simulink subsystem "SSCFuelCell"  (R2025b)
settings: Solver=VariableStepAuto  StartTime=0.0  StopTime=10.0  RelTol=1e-3
undefined symbols (not defined in the file): anode_tube_D, cathode_tube_D, comp_rpm_TLU, coolant_num_layers, coolant_num_passes, coolant_tube_D, coolant_w_channels, env_p, env_T, f_fc_voltage, N2_T, radiator_air_area_fins, radiator_air_area_primary, radiator_eta_fin, radiator_N_tubes, radiator_rho, radiator_t_wall, radiator_tube_H, radiator_W, stack_area, stack_iL, stack_mea_rho, stack_num_cells, stack_num_channels, stack_t_gdl, stack_t_membrane, stack_w_channels
libraries: fl_lib x100, nesl_utility x20, slpidlib x2
(part 3 of 3)

== system SSCFuelCell/Recirculation ==
  Constant Volume Chamber (MA) : fl_lib/Moist Air/Elements/Constant Volume Chamber (MA)  volume=0.05^3 m^3  num_ports=foundation.enum.num_ports.three  area_A=pi*anode_tube_D^2/4 m^2  area_B=pi*anode_tube_D^2/4 m^2  area_C=pi*anode_tube_D^2/4 m^2  area_D=0.01 m^2  RH_ws=1  time_constant_cond=1e-3 s  time_constant_evap=1e-3 s  fraction_entrained=1  moisture_trace_gas_source=foundation.enum.moisture_trace_gas_source.none  moisture_source_spec=foundation.enum.MoistureSourceSpec.WaterVapor  vapor_from_liquid=false  moisture_mass_flow=0 kg/s  moisture_temperature_spec=foundation.enum.temperature_spec.atmospheric  moisture_temperature=293.15 K  trace_gas_mass_flow=0 kg/s  trace_gas_temperature_spec=foundation.enum.temperature_spec.atmospheric  trace_gas_temperature=293.15 K  p_init=env_p MPa  p_init_priority=foundation.enum.Priority.High  T_init=env_T degC  T_init_priority=foundation.enum.Priority.High  humidity_spec=foundation.enum.HumiditySpec.RelativeHumidity  RH_init=0  RH_init_priority=foundation.enum.Priority.High  x_w_init=0  x_w_init_priority=foundation.enum.Priority.None  y_w_init=0  y_w_init_priority=foundation.enum.Priority.None  HR_init=0  HR_init_priority=foundation.enum.Priority.None  Tw_init=287 K  Tw_init_priority=foundation.enum.Priority.High  trace_gas_spec=foundation.enum.trace_gas_spec.mole_fraction  x_g_init=0  x_g_init_priority=foundation.enum.Priority.None  y_g_init=tank_yH2  y_g_init_priority=foundation.enum.Priority.High  r_d_init=0  r_d_init_priority=foundation.enum.Priority.High
      settings: InternalSimscapePortConfiguration="{\"Bottom\":[],\"Left\":[{\"id\":\"A\",\"label\":\"A\",\"type\":\"foundation.moist_air.moist_air\"},{\"id\":\"B\",\"label\":\"B\",\"type\":\"foundation.moist_air.moist_air\"},{\"id\":\"C\",\"label\":\"C\",\"type\":\"foundation.moist_air.moist_air\"}],\"Right\":[{\"id\":\"W\",\"label\":\"W\",\"type\":\"output\"},{\"id\":\"F\",\"label\":\"F\",\"type\":\"output\"},{\"id\":\"H\",\"label\":\"H\",\"type\":\"foundation.thermal.thermal\"}],\"Top\":[]}"
  Controlled Mass Flow Rate Source (MA) : fl_lib/Moist Air/Sources/Flow Rate Source (MA)  source_type=foundation.enum.constant_controlled.controlled  flow_type=foundation.enum.mass_volumetric_flow.mass  mass_flow=0 kg/s  volumetric_flow=0 m^3/s  volumetric_flow_conditions=foundation.enum.volumetric_flow_conditions.actual  p_std=0.101325 MPa  T_std=20 degC  RH_std=0.65  power_spec=foundation.enum.power_spec.isentropic  area_A=pi*anode_tube_D^2/4 m^2  area_B=pi*anode_tube_D^2/4 m^2
      settings: InternalSimscapePortConfiguration="{\"Bottom\":[],\"Left\":[{\"id\":\"A\",\"label\":\"A\",\"type\":\"foundation.moist_air.moist_air\"},{\"id\":\"M\",\"label\":\"M\",\"type\":\"input\"}],\"Right\":[{\"id\":\"B\",\"label\":\"B\",\"type\":\"foundation.moist_air.moist_air\"}],\"Top\":[]}"
  Feedforward Control : Subsystem
  Max Flow : fl_lib/Physical Signals/Functions/PS Gain  gain=0.01 kg/s
  Perfect Insulator : fl_lib/Thermal/Thermal Elements/Perfect Insulator  T_specify=off  T_priority=None  T=0 K  T_nominal_specify=off  T_nominal_value=1  T_nominal_unit=K
  Simulink-PS Converter : nesl_utility/Simulink-PS Converter  PhysicalDomain=network_engine_domain  SubClassName=ps_input  LeftPortType=input  RightPortType=output  PseudoPeriodic=off  Frequencies=[]  NoiseDistribution=none  NoiseParameters=[]  Unit=1  AffineConversion=off  FilteringAndDerivatives=provide  SimscapeFilterOrder=1  InputFilterTimeConstant=0.001  UdotUserProvided=0
  A : PMIOPort  Side=Left
  B : PMIOPort  Port=2  Side=Right
  R : PMIOPort  Port=3  Side=Right
  wires:
  [i_stack] -> Feedforward Control/1(i)
  Feedforward Control/1(cmd) -> Simulink-PS Converter/1
  connections:
  Perfect Insulator/LConn1 -- Constant Volume Chamber (MA)/RConn3
  Controlled Mass Flow Rate Source (MA)/RConn1 -- Constant Volume Chamber (MA)/LConn2
  A/RConn1 -- Constant Volume Chamber (MA)/LConn1
  B/RConn1 -- Constant Volume Chamber (MA)/LConn3
  R/RConn1 -- Controlled Mass Flow Rate Source (MA)/LConn1
  Max Flow/RConn1 -- Controlled Mass Flow Rate Source (MA)/LConn2
  Simulink-PS Converter/RConn1 -- Max Flow/LConn1

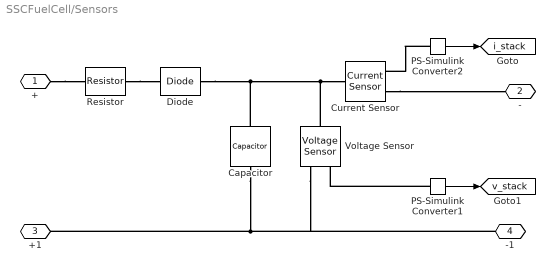
== system SSCFuelCell/Sensors ==
  Capacitor : fl_lib/Electrical/Electrical Elements/Capacitor  c=1e-6 F  r=1e-6 Ohm  g=0 1/Ohm  i_specify=off  i_priority=None  i=0 A  i_nominal_specify=off  i_nominal_value=1  i_nominal_unit=A  v_specify=off  v_priority=None  v=0 V  v_nominal_specify=off  v_nominal_value=1  v_nominal_unit=V  vc_specify=on  vc_priority=High  vc=f_fc_voltage(1) V  vc_nominal_specify=off  vc_nominal_value=1  vc_nominal_unit=V
  Current Sensor : fl_lib/Electrical/Electrical Sensors/Current Sensor
  Diode : fl_lib/Electrical/Electrical Elements/Diode  Vf=0.6 V  Ron=0.3 Ohm  Goff=1e-8 1/Ohm  i_specify=off  i_priority=None  i=0 A  i_nominal_specify=off  i_nominal_value=1  i_nominal_unit=A  v_specify=off  v_priority=None  v=0 V  v_nominal_specify=off  v_nominal_value=1  v_nominal_unit=V
  PS-Simulink Converter1 : nesl_utility/PS-Simulink Converter  PhysicalDomain=network_engine_domain  SubClassName=ps_output  LeftPortType=input  RightPortType=output  PseudoPeriodic=off  Frequencies=[]  VectorFormat=1-D array  Unit=V  AffineConversion=off
  PS-Simulink Converter2 : nesl_utility/PS-Simulink Converter  PhysicalDomain=network_engine_domain  SubClassName=ps_output  LeftPortType=input  RightPortType=output  PseudoPeriodic=off  Frequencies=[]  VectorFormat=1-D array  Unit=A  AffineConversion=off
  Resistor : fl_lib/Electrical/Electrical Elements/Resistor  R=1e-3 Ohm  i_specify=off  i_priority=None  i=0 A  i_nominal_specify=off  i_nominal_value=1  i_nominal_unit=A  v_specify=off  v_priority=None  v=0 V  v_nominal_specify=off  v_nominal_value=1  v_nominal_unit=V
  Voltage Sensor : fl_lib/Electrical/Electrical Sensors/Voltage Sensor
  + : PMIOPort  Side=Left
  - : PMIOPort  Port=2  Side=Right
  +1 : PMIOPort  Port=3  Side=Left
  -1 : PMIOPort  Port=4  Side=Right
  tag scope: i_stack=global, v_stack=global
  wires:
  PS-Simulink Converter1/1 -> [v_stack]
  PS-Simulink Converter2/1 -> [i_stack]
  connections:
  Capacitor/RConn1 -- -1/RConn1 -- Voltage Sensor/RConn2 -- +1/RConn1
  Capacitor/LConn1 -- Diode/RConn1 -- Current Sensor/LConn1 -- Voltage Sensor/LConn1
  +/RConn1 -- Resistor/LConn1
  Current Sensor/RConn2 -- -/RConn1
  PS-Simulink Converter1/LConn1 -- Voltage Sensor/RConn1
  Resistor/RConn1 -- Diode/LConn1
  PS-Simulink Converter2/LConn1 -- Current Sensor/RConn1

== system SSCFuelCell/Anode Humidifier/Proportional Control ==
  RH_set : Inport
  RH_meas : Inport  Port=2
  Gain : Gain  Gain=0.1
  Saturation : Saturate  UpperLimit=inf  LowerLimit=0  ZeroCross=off
  Sum : Sum  Inputs=|+-
  Transfer Fcn : TransferFcn  Denominator=[1 1]
  Mw : Outport
  wires:
  Saturation/1 -> Transfer Fcn/1
  RH_meas/1 -> Sum/2
  RH_set/1 -> Sum/1
  Sum/1 -> Gain/1
  Gain/1 -> Saturation/1
  Transfer Fcn/1 -> Mw/1

== system SSCFuelCell/Cathode Humidifier/Proportional Control ==
  RH_set : Inport
  RH_meas : Inport  Port=2
  Gain : Gain  Gain=0.1
  Saturation : Saturate  UpperLimit=inf  LowerLimit=0  ZeroCross=off
  Sum : Sum  Inputs=|+-
  Transfer Fcn : TransferFcn  Denominator=[1 1]
  Mw : Outport
  wires:
  Saturation/1 -> Transfer Fcn/1
  Gain/1 -> Saturation/1
  Transfer Fcn/1 -> Mw/1
  RH_meas/1 -> Sum/2
  Sum/1 -> Gain/1
  RH_set/1 -> Sum/1

== system SSCFuelCell/Cathode Exhaust/Pressure Relief Valve ==
  Absolute Reference (MA) : fl_lib/Moist Air/Elements/Absolute Reference (MA)
  PS Add : fl_lib/Physical Signals/Functions/PS Add
  PS Constant : fl_lib/Physical Signals/Sources/PS Constant  constant=r_min^2
  PS Gain : fl_lib/Physical Signals/Functions/PS Gain  gain=(r_max^2 - r_min^2)/p_range 1/MPa
  PS Gain1 : fl_lib/Physical Signals/Functions/PS Gain  gain=pi*D^2/4 m^2
  PS Subtract : fl_lib/Physical Signals/Functions/PS Subtract
  Pressure & Temperature Sensor (MA) : fl_lib/Moist Air/Sensors/Pressure & Temperature Sensor (MA)  reference=foundation.enum.MeasurementReference.difference  pressure=true  pressure_spec=foundation.enum.PressureMeasementSpec.Absolute  temperature=true
      settings: InternalSimscapePortConfiguration="{\"Bottom\":[{\"id\":\"T\",\"label\":\"T\",\"type\":\"output\"}],\"Left\":[{\"id\":\"A\",\"label\":\"A\",\"type\":\"foundation.moist_air.moist_air\"}],\"Right\":[{\"id\":\"B\",\"label\":\"B\",\"type\":\"foundation.moist_air.moist_air\"},{\"id\":\"P\",\"label\":\"P\",\"type\":\"output\"}],\"Top\":[]}"
  Valve : fl_lib/Moist Air/Elements/Local Restriction (MA)  restriction_type=foundation.enum.restriction_type.variable  restriction_area=0.001 m^2  min_area=pi*(r_min*D)^2/4 m^2  max_area=pi*(r_max*D)^2/4 m^2  area=pi*D^2/4 m^2  Cd=0.64  B_lam=0.999
  A : PMIOPort  Side=Left
  B : PMIOPort  Port=2  Side=Right
  p_set : PMIOPort  Port=3  Side=Left
  connections:
  PS Add/RConn1 -- PS Gain1/LConn1
  PS Gain/LConn1 -- PS Subtract/RConn1
  PS Gain1/RConn1 -- Valve/LConn2
  Absolute Reference (MA)/LConn1 -- Pressure & Temperature Sensor (MA)/RConn1
  Valve/RConn1 -- B/RConn1
  Valve/LConn1 -- A/RConn1 -- Pressure & Temperature Sensor (MA)/LConn1
  PS Gain/RConn1 -- PS Add/LConn1
  PS Add/LConn2 -- PS Constant/RConn1
  Pressure & Temperature Sensor (MA)/RConn2 -- PS Subtract/LConn1
  p_set/RConn1 -- PS Subtract/LConn2

== system SSCFuelCell/Cooling System/Coolant Tank ==
  Coolant Volume : fl_lib/Thermal Liquid/Elements/Translational Mechanical Converter (TL)  mech_orientation=foundation.enum.MechOrientationTranslational.Positive  displacement_spec=foundation.enum.DisplacementSpec.Calculate  x0=x_init m  interface_area=A m^2  dead_volume=A * 0.001 m^3  environment_spec=foundation.enum.pressure_spec.atmospheric  environment_pressure=0.101325 MPa  dynamic_compressibility=simscape.enum.onoff.off  p0=env_p MPa  T0=env_T degC  p_nominal=0.101325 MPa  T_nominal=293.15 K
      settings: InternalSimscapePortConfiguration="{\"Bottom\":[],\"Left\":[{\"id\":\"A\",\"label\":\"A\",\"type\":\"foundation.thermal_liquid.thermal_liquid\"},{\"id\":\"C\",\"label\":\"C\",\"type\":\"foundation.mechanical.translational.translational\"},{\"id\":\"H\",\"label\":\"H\",\"type\":\"foundation.thermal.thermal\"}],\"Right\":[{\"id\":\"R\",\"label\":\"R\",\"type\":\"foundation.mechanical.translational.translational\"}],\"Top\":[]}"
  Mechanical Translational Reference : fl_lib/Mechanical/Translational Elements/Mechanical Translational Reference
  Perfect Insulator : fl_lib/Thermal/Thermal Elements/Perfect Insulator  T_specify=off  T_priority=None  T=0 K  T_nominal_specify=off  T_nominal_value=1  T_nominal_unit=K
  Translational Free End : fl_lib/Mechanical/Translational Elements/Translational Free End  v_specify=off  v_priority=None  v=0 m/s  v_nominal_specify=off  v_nominal_value=1  v_nominal_unit=m/s
      settings: InternalSimscapePortConfiguration="{\"Bottom\":[],\"Left\":[{\"id\":\"V\",\"label\":\"\",\"type\":\"foundation.mechanical.translational.translational\"}],\"Right\":[],\"Top\":[]}"
  T : PMIOPort  Side=Right
  connections:
  Coolant Volume/LConn1 -- T/RConn1
  Mechanical Translational Reference/LConn1 -- Coolant Volume/LConn2
  Translational Free End/LConn1 -- Coolant Volume/RConn1
  Perfect Insulator/LConn1 -- Coolant Volume/LConn3

== system SSCFuelCell/Cooling System/Pump Control ==
  T_set : Inport
  T_meas : Inport  Port=2
  Control Signals : Scope  NumInputPorts=2
      settings: Title=Stack Temperature (degC)  ActiveDisplayYMinimum=12.33618  ActiveDisplayYMaximum=88.97437
  Mux : Mux  Inputs=2
  Mux1 : Mux  Inputs=2
  PID Controller : slpidlib/PID Controller  Controller=PI  Form=Ideal  TimeDomain=Continuous-time  UseExternalTs=off  SampleTime=-1  IntegratorMethod=Forward Euler  FilterMethod=Forward Euler  ControllerParametersSource=internal  P=0.1  I=0.01  UseKiTs=off  D=0  UseExternalDerivativeSource=off  N=100  UseFilter=on  TunerSelectOption=Transfer Function Based (PID Tuner App)  InitialConditionSource=internal  InitialConditionForIntegrator=0  InitialConditionForFilter=0  DifferentiatorICPrevScaledInput=0  ExternalReset=none  TrackingMode=off  Kt=1  LimitOutput=on  SatLimitsSource=internal  UpperSaturationLimit=1  LowerSaturationLimit=0  LinearizeAsGain=on  AntiWindupMode=back-calculation  Kb=0.1  LimitIntegrator=off  UpperIntegratorSaturationLimit=inf  LowerIntegratorSaturationLimit=-inf  POutMin=[]  POutMax=[]  IOutMin=[]  IOutMax=[]  DOutMin=[]  DOutMax=[]  NOutMin=[]  NOutMax=[]  SumOutMin=[]  SumOutMax=[]  SaturationOutMin=[]  SaturationOutMax=[]  PParamMin=[]  PParamMax=[]  IParamMin=[]  IParamMax=[]  DParamMin=[]  DParamMax=[]  NParamMin=[]  NParamMax=[]  KbParamMin=[]  KbParamMax=[]  KtParamMin=[]  KtParamMax=[]  KbOutMin=[]  KbOutMax=[]  KtOutMin=[]  KtOutMax=[]  IntegratorOutMin=[]  IntegratorOutMax=[]  FilterOutMin=[]  FilterOutMax=[]  SumI1OutMin=[]  SumI1OutMax=[]  SumI2OutMin=[]  SumI2OutMax=[]  SumI3OutMin=[]  SumI3OutMax=[]  SumI4OutMin=[]  SumI4OutMax=[]  SumDOutMin=[]  SumDOutMax=[]  DifferentiatorOutMin=[]  DifferentiatorOutMax=[]  FilterDiffOutCoefMin=[]  FilterDiffOutCoefMax=[]  ReciprocalOutMin=[]  ReciprocalOutMax=[]  SumDenOutMin=[]  SumDenOutMax=[]  SumNumOutMin=[]  SumNumOutMax=[]  DivideOutMin=[]  DivideOutMax=[]  UdiffTsProdOutMin=[]  UdiffTsProdOutMax=[]  NTsProdOutMin=[]  NTsProdOutMax=[]  UintegralTsProdOutMin=[]  UintegralTsProdOutMax=[]  UngainTsProdOutMin=[]  UngainTsProdOutMax=[]  ClampingZeroOutDataTypeStr=Inherit: Inherit via back propagation  ClampingZeroOutMin=[]  ClampingZeroOutMax=[]  FilterDenConstantOutDataTypeStr=Inherit: Inherit via back propagation  FilterDenConstantOutMin=[]  FilterDenConstantOutMax=[]  PCopyOutDataTypeStr=Inherit: Inherit via back propagation  PCopyOutMin=[]  PCopyOutMax=[]  NCopyOutDataTypeStr=Inherit: Inherit via back propagation  NCopyOutMin=[]  NCopyOutMax=[]  IntegratorContinuousStateAttributes=''  IntegratorStateMustResolveToSignalObject=off  IntegratorRTWStateStorageClass=Auto  FilterContinuousStateAttributes=''  FilterStateMustResolveToSignalObject=off  FilterRTWStateStorageClass=Auto  ParallelPVariant=Passthrough  IdealPVariant=InternalParameters  IVariant=InternalParameters  DVariant=Disabled  IntegratorVariant=Continuous  SatVariant=Enabled  AWVariant=BackCalculation  PCopyVariant=Disabled  TRVariant=Disabled  FdbkBlocksVariant=Forward  IdealPFdbkVariant=Disabled  SatFdbkVariant=Disabled  DerivativeFilterVariant=Disabled  NVariant=Disabled  NCopyVariant=Disabled_SignalSpec  FilterICVariant=Disabled  IntegratorICVariant=InternalICs  ExternalResetVariant=Disabled  TRSumVariant=Passthrough  SumFdbkVariant=Disabled  SumVariant=Sum_PI  TsampFilterVariant=InternalTs  TsampNgainVariant=Passthrough  TsampIntegralVariant=Disabled_SignalSpec  ExternalSaturationOutDataTypeStr=Inherit: Same as second input  DerivativeSourceVariant=Disabled  PreIntVariant=InternalPreInt
  Sum : Sum  Inputs=|-+
  Transfer Fcn : TransferFcn  Denominator=[2 1]
  cmd : Outport
  wires:
  Transfer Fcn/1 -> Mux1/2, cmd/1
  T_set/1 -> Mux/1, Sum/1
  T_meas/1 -> Mux/2, Sum/2
  Sum/1 -> PID Controller/1
  PID Controller/1 -> Mux1/1, Transfer Fcn/1
  Mux/1 -> Control Signals/1
  Mux1/1 -> Control Signals/2

== system SSCFuelCell/Cooling System/Sensors ==
  Abs : Abs  ZeroCross=off  SaturateOnIntegerOverflow=off
  Average Efficiency : fl_lib/Physical Signals/Sources/PS Constant  constant=0.9
  PS Divide : fl_lib/Physical Signals/Functions/PS Divide
  PS Product : fl_lib/Physical Signals/Functions/PS Product
  PS-Simulink Converter : nesl_utility/PS-Simulink Converter  PhysicalDomain=network_engine_domain  SubClassName=ps_output  LeftPortType=input  RightPortType=output  PseudoPeriodic=off  Frequencies=[]  VectorFormat=1-D array  Unit=inherit  AffineConversion=off
  Pressure & Temperature Sensor (TL) : fl_lib/Thermal Liquid/Sensors/Pressure & Temperature Sensor (TL)  reference=foundation.enum.MeasurementReference.difference  pressure=true  pressure_spec=foundation.enum.PressureMeasementSpec.Absolute  temperature=true
      settings: InternalSimscapePortConfiguration="{\"Bottom\":[{\"id\":\"T\",\"label\":\"T\",\"type\":\"output\"}],\"Left\":[{\"id\":\"A\",\"label\":\"A\",\"type\":\"foundation.thermal_liquid.thermal_liquid\"}],\"Right\":[{\"id\":\"B\",\"label\":\"B\",\"type\":\"foundation.thermal_liquid.thermal_liquid\"},{\"id\":\"P\",\"label\":\"P\",\"type\":\"output\"}],\"Top\":[]}"
  Volumetric Flow Rate Sensor (TL) : fl_lib/Thermal Liquid/Sensors/Flow Rate Sensor (TL)  mass_flow_measure=false  volumetric_flow_measure=true  energy_flow_measure=false
      settings: InternalSimscapePortConfiguration="{\"Bottom\":[],\"Left\":[{\"id\":\"A\",\"label\":\"A\",\"type\":\"foundation.thermal_liquid.thermal_liquid\"}],\"Right\":[{\"id\":\"B\",\"label\":\"B\",\"type\":\"foundation.thermal_liquid.thermal_liquid\"},{\"id\":\"V\",\"label\":\"V\",\"type\":\"output\"}],\"Top\":[]}"
  B : PMIOPort  Side=Left
  A_P : PMIOPort  Port=2  Side=Right
  A : PMIOPort  Port=3  Side=Right
  Power : Outport
  wires:
  Abs/1 -> Power/1
  PS-Simulink Converter/1 -> Abs/1
  connections:
  A/RConn1 -- Volumetric Flow Rate Sensor (TL)/LConn1
  A_P/RConn1 -- Pressure & Temperature Sensor (TL)/LConn1
  PS-Simulink Converter/LConn1 -- PS Divide/RConn1
  Average Efficiency/RConn1 -- PS Divide/LConn2
  PS Divide/LConn1 -- PS Product/RConn1
  Volumetric Flow Rate Sensor (TL)/RConn2 -- PS Product/LConn2
  PS Product/LConn1 -- Pressure & Temperature Sensor (TL)/RConn2
  B/RConn1 -- Volumetric Flow Rate Sensor (TL)/RConn1 -- Pressure & Temperature Sensor (TL)/RConn1

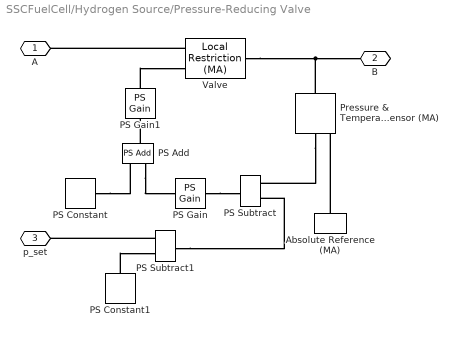
== system SSCFuelCell/Hydrogen Source/Pressure-Reducing Valve ==
  Absolute Reference (MA) : fl_lib/Moist Air/Elements/Absolute Reference (MA)
  PS Add : fl_lib/Physical Signals/Functions/PS Add
  PS Constant : fl_lib/Physical Signals/Sources/PS Constant  constant=r_max^2
  PS Constant1 : fl_lib/Physical Signals/Sources/PS Constant  constant=p_range MPa
  PS Gain : fl_lib/Physical Signals/Functions/PS Gain  gain=(r_min^2 - r_max^2)/p_range 1/MPa
  PS Gain1 : fl_lib/Physical Signals/Functions/PS Gain  gain=pi*D^2/4 m^2
  PS Subtract : fl_lib/Physical Signals/Functions/PS Subtract
  PS Subtract1 : fl_lib/Physical Signals/Functions/PS Subtract
  Pressure & Temperature Sensor (MA) : fl_lib/Moist Air/Sensors/Pressure & Temperature Sensor (MA)  reference=foundation.enum.MeasurementReference.difference  pressure=true  pressure_spec=foundation.enum.PressureMeasementSpec.Absolute  temperature=true
      settings: InternalSimscapePortConfiguration="{\"Bottom\":[{\"id\":\"T\",\"label\":\"T\",\"type\":\"output\"}],\"Left\":[{\"id\":\"A\",\"label\":\"A\",\"type\":\"foundation.moist_air.moist_air\"}],\"Right\":[{\"id\":\"B\",\"label\":\"B\",\"type\":\"foundation.moist_air.moist_air\"},{\"id\":\"P\",\"label\":\"P\",\"type\":\"output\"}],\"Top\":[]}"
  Valve : fl_lib/Moist Air/Elements/Local Restriction (MA)  restriction_type=foundation.enum.restriction_type.variable  restriction_area=0.001 m^2  min_area=pi*(r_min*D)^2/4 m^2  max_area=pi*(r_max*D)^2/4 m^2  area=pi*D^2/4 m^2  Cd=0.64  B_lam=0.999
  A : PMIOPort  Side=Left
  B : PMIOPort  Port=2  Side=Right
  p_set : PMIOPort  Port=3  Side=Left
  connections:
  PS Constant1/RConn1 -- PS Subtract1/LConn2
  PS Subtract1/LConn1 -- p_set/RConn1
  PS Subtract1/RConn1 -- PS Subtract/LConn2
  PS Constant/RConn1 -- PS Add/LConn1
  PS Add/LConn2 -- PS Gain/RConn1
  PS Add/RConn1 -- PS Gain1/LConn1
  PS Gain/LConn1 -- PS Subtract/RConn1
  Pressure & Temperature Sensor (MA)/RConn2 -- PS Subtract/LConn1
  PS Gain1/RConn1 -- Valve/LConn2
  Absolute Reference (MA)/LConn1 -- Pressure & Temperature Sensor (MA)/RConn1
  Pressure & Temperature Sensor (MA)/LConn1 -- B/RConn1 -- Valve/RConn1
  Valve/LConn1 -- A/RConn1

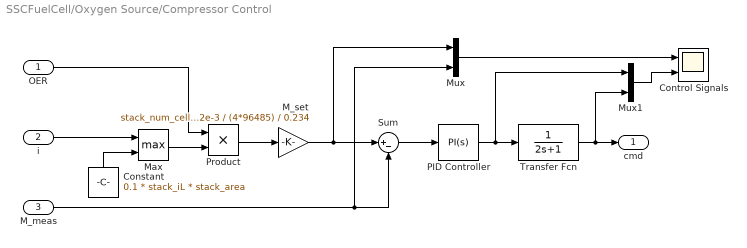
== system SSCFuelCell/Oxygen Source/Compressor Control ==
  OER : Inport
  i : Inport  Port=2
  M_meas : Inport  Port=3
  Constant : Constant  Value=0.1 * stack_iL * stack_area
  Control Signals : Scope  NumInputPorts=2
      settings: Title=Mass Flow Rate (kg/s)  ActiveDisplayYMinimum=-0.01736  ActiveDisplayYMaximum=0.15625  DataLoggingVariableName=ScopeData2
  M_set : Gain  Gain=stack_num_cells * 32e-3 / (4*96485) / 0.234
  Max : MinMax  Function=max  Inputs=2  ZeroCross=off
  Mux : Mux  Inputs=2
  Mux1 : Mux  Inputs=2
  PID Controller : slpidlib/PID Controller  Controller=PI  Form=Ideal  TimeDomain=Continuous-time  UseExternalTs=off  SampleTime=-1  IntegratorMethod=Forward Euler  FilterMethod=Forward Euler  ControllerParametersSource=internal  P=5  I=0.5  UseKiTs=off  D=0  UseExternalDerivativeSource=off  N=100  UseFilter=on  TunerSelectOption=Transfer Function Based (PID Tuner App)  InitialConditionSource=internal  InitialConditionForIntegrator=0  InitialConditionForFilter=0  DifferentiatorICPrevScaledInput=0  ExternalReset=none  TrackingMode=off  Kt=1  LimitOutput=on  SatLimitsSource=internal  UpperSaturationLimit=1  LowerSaturationLimit=0  LinearizeAsGain=on  AntiWindupMode=back-calculation  Kb=1  LimitIntegrator=off  UpperIntegratorSaturationLimit=inf  LowerIntegratorSaturationLimit=-inf  POutMin=[]  POutMax=[]  IOutMin=[]  IOutMax=[]  DOutMin=[]  DOutMax=[]  NOutMin=[]  NOutMax=[]  SumOutMin=[]  SumOutMax=[]  SaturationOutMin=[]  SaturationOutMax=[]  PParamMin=[]  PParamMax=[]  IParamMin=[]  IParamMax=[]  DParamMin=[]  DParamMax=[]  NParamMin=[]  NParamMax=[]  KbParamMin=[]  KbParamMax=[]  KtParamMin=[]  KtParamMax=[]  KbOutMin=[]  KbOutMax=[]  KtOutMin=[]  KtOutMax=[]  IntegratorOutMin=[]  IntegratorOutMax=[]  FilterOutMin=[]  FilterOutMax=[]  SumI1OutMin=[]  SumI1OutMax=[]  SumI2OutMin=[]  SumI2OutMax=[]  SumI3OutMin=[]  SumI3OutMax=[]  SumI4OutMin=[]  SumI4OutMax=[]  SumDOutMin=[]  SumDOutMax=[]  DifferentiatorOutMin=[]  DifferentiatorOutMax=[]  FilterDiffOutCoefMin=[]  FilterDiffOutCoefMax=[]  ReciprocalOutMin=[]  ReciprocalOutMax=[]  SumDenOutMin=[]  SumDenOutMax=[]  SumNumOutMin=[]  SumNumOutMax=[]  DivideOutMin=[]  DivideOutMax=[]  UdiffTsProdOutMin=[]  UdiffTsProdOutMax=[]  NTsProdOutMin=[]  NTsProdOutMax=[]  UintegralTsProdOutMin=[]  UintegralTsProdOutMax=[]  UngainTsProdOutMin=[]  UngainTsProdOutMax=[]  ClampingZeroOutDataTypeStr=Inherit: Inherit via back propagation  ClampingZeroOutMin=[]  ClampingZeroOutMax=[]  FilterDenConstantOutDataTypeStr=Inherit: Inherit via back propagation  FilterDenConstantOutMin=[]  FilterDenConstantOutMax=[]  PCopyOutDataTypeStr=Inherit: Inherit via back propagation  PCopyOutMin=[]  PCopyOutMax=[]  NCopyOutDataTypeStr=Inherit: Inherit via back propagation  NCopyOutMin=[]  NCopyOutMax=[]  IntegratorContinuousStateAttributes=''  IntegratorStateMustResolveToSignalObject=off  IntegratorRTWStateStorageClass=Auto  FilterContinuousStateAttributes=''  FilterStateMustResolveToSignalObject=off  FilterRTWStateStorageClass=Auto  ParallelPVariant=Passthrough  IdealPVariant=InternalParameters  IVariant=InternalParameters  DVariant=Disabled  IntegratorVariant=Continuous  SatVariant=Enabled  AWVariant=BackCalculation  PCopyVariant=Disabled  TRVariant=Disabled  FdbkBlocksVariant=Forward  IdealPFdbkVariant=Disabled  SatFdbkVariant=Disabled  DerivativeFilterVariant=Disabled  NVariant=Disabled  NCopyVariant=Disabled_SignalSpec  FilterICVariant=Disabled  IntegratorICVariant=InternalICs  ExternalResetVariant=Disabled  TRSumVariant=Passthrough  SumFdbkVariant=Disabled  SumVariant=Sum_PI  TsampFilterVariant=InternalTs  TsampNgainVariant=Passthrough  TsampIntegralVariant=Disabled_SignalSpec  ExternalSaturationOutDataTypeStr=Inherit: Same as second input  DerivativeSourceVariant=Disabled  PreIntVariant=InternalPreInt
  Product : Product
  Sum : Sum  Inputs=|+-
  Transfer Fcn : TransferFcn  Denominator=[2 1]
  cmd : Outport
  wires:
  OER/1 -> Product/1
  Constant/1 -> Max/2
  i/1 -> Max/1
  Max/1 -> Product/2
  PID Controller/1 -> Mux1/1, Transfer Fcn/1
  Sum/1 -> PID Controller/1
  M_set/1 -> Sum/1, Mux/1
  Product/1 -> M_set/1
  M_meas/1 -> Mux/2, Sum/2
  Transfer Fcn/1 -> Mux1/2, cmd/1
  Mux/1 -> Control Signals/1
  Mux1/1 -> Control Signals/2

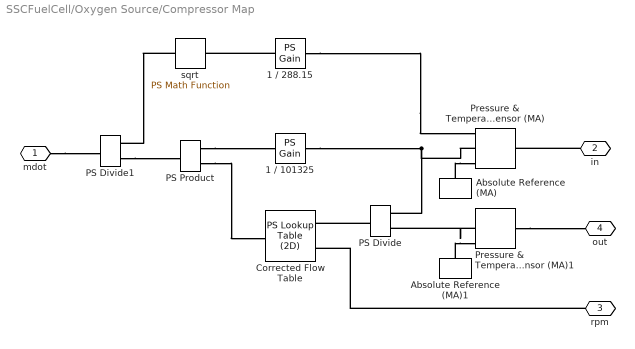
== system SSCFuelCell/Oxygen Source/Compressor Map ==
  1 / 101325 : fl_lib/Physical Signals/Functions/PS Gain  gain=1 / 101325 1/Pa
  1 / 288.15 : fl_lib/Physical Signals/Functions/PS Gain  gain=1 / 288.15 1/K
  Absolute Reference (MA) : fl_lib/Moist Air/Elements/Absolute Reference (MA)
  Absolute Reference (MA)1 : fl_lib/Moist Air/Elements/Absolute Reference (MA)
  Corrected Flow Table : fl_lib/Physical Signals/Lookup Tables/PS Lookup Table (2D)  x1=comp_p_ratio_TLU Pa/Pa  x2=comp_rpm_TLU rpm  f=comp_mdot_corr_TLU kg/s  interp_method=simscape.enum.interpolation.linear  extrap_method=simscape.enum.extrapolation.nearest
  PS Divide : fl_lib/Physical Signals/Functions/PS Divide
  PS Divide1 : fl_lib/Physical Signals/Functions/PS Divide
  PS Product : fl_lib/Physical Signals/Functions/PS Product
  Pressure & Temperature Sensor (MA) : fl_lib/Moist Air/Sensors/Pressure & Temperature Sensor (MA)  reference=foundation.enum.MeasurementReference.difference  pressure=true  pressure_spec=foundation.enum.PressureMeasementSpec.Absolute  temperature=true
      settings: InternalSimscapePortConfiguration="{\"Bottom\":[{\"id\":\"T\",\"label\":\"T\",\"type\":\"output\"}],\"Left\":[{\"id\":\"A\",\"label\":\"A\",\"type\":\"foundation.moist_air.moist_air\"}],\"Right\":[{\"id\":\"B\",\"label\":\"B\",\"type\":\"foundation.moist_air.moist_air\"},{\"id\":\"P\",\"label\":\"P\",\"type\":\"output\"}],\"Top\":[]}"
  Pressure & Temperature Sensor (MA)1 : fl_lib/Moist Air/Sensors/Pressure & Temperature Sensor (MA)  reference=foundation.enum.MeasurementReference.difference  pressure=true  pressure_spec=foundation.enum.PressureMeasementSpec.Absolute  temperature=true
      settings: InternalSimscapePortConfiguration="{\"Bottom\":[{\"id\":\"T\",\"label\":\"T\",\"type\":\"output\"}],\"Left\":[{\"id\":\"A\",\"label\":\"A\",\"type\":\"foundation.moist_air.moist_air\"}],\"Right\":[{\"id\":\"B\",\"label\":\"B\",\"type\":\"foundation.moist_air.moist_air\"},{\"id\":\"P\",\"label\":\"P\",\"type\":\"output\"}],\"Top\":[]}"
  sqrt : fl_lib/Physical Signals/Functions/PS Math Function  fcn_choice=foundation.enum.math_function.sqrt  v=1
  mdot : PMIOPort  Side=Left
  in : PMIOPort  Port=2  Side=Right
  rpm : PMIOPort  Port=3  Side=Right
  out : PMIOPort  Port=4  Side=Right
  connections:
  Pressure & Temperature Sensor (MA)1/LConn1 -- out/RConn1
  Absolute Reference (MA)/LConn1 -- Pressure & Temperature Sensor (MA)/RConn1
  in/RConn1 -- Pressure & Temperature Sensor (MA)/LConn1
  1 / 101325/LConn1 -- Pressure & Temperature Sensor (MA)/RConn2 -- PS Divide/LConn2
  rpm/RConn1 -- Corrected Flow Table/LConn2
  PS Divide/RConn1 -- Corrected Flow Table/LConn1
  1 / 288.15/LConn1 -- Pressure & Temperature Sensor (MA)/RConn3
  PS Product/LConn1 -- 1 / 101325/RConn1
  PS Product/LConn2 -- Corrected Flow Table/RConn1
  PS Divide1/LConn1 -- PS Product/RConn1
  1 / 288.15/RConn1 -- sqrt/LConn1
  sqrt/RConn1 -- PS Divide1/LConn2
  mdot/RConn1 -- PS Divide1/RConn1
  Absolute Reference (MA)1/LConn1 -- Pressure & Temperature Sensor (MA)1/RConn1
  Pressure & Temperature Sensor (MA)1/RConn2 -- PS Divide/LConn1

== system SSCFuelCell/Oxygen Source/Sensors ==
  Abs : Abs  ZeroCross=off  SaturateOnIntegerOverflow=off
  Average Efficiency : fl_lib/Physical Signals/Sources/PS Constant  constant=0.9
  PS Divide : fl_lib/Physical Signals/Functions/PS Divide
  PS Product : fl_lib/Physical Signals/Functions/PS Product
  PS-Simulink Converter : nesl_utility/PS-Simulink Converter  PhysicalDomain=network_engine_domain  SubClassName=ps_output  LeftPortType=input  RightPortType=output  PseudoPeriodic=off  Frequencies=[]  VectorFormat=1-D array  Unit=inherit  AffineConversion=off
  Pressure & Temperature Sensor (MA) : fl_lib/Moist Air/Sensors/Pressure & Temperature Sensor (MA)  reference=foundation.enum.MeasurementReference.difference  pressure=true  pressure_spec=foundation.enum.PressureMeasementSpec.Absolute  temperature=true
      settings: InternalSimscapePortConfiguration="{\"Bottom\":[{\"id\":\"T\",\"label\":\"T\",\"type\":\"output\"}],\"Left\":[{\"id\":\"A\",\"label\":\"A\",\"type\":\"foundation.moist_air.moist_air\"}],\"Right\":[{\"id\":\"B\",\"label\":\"B\",\"type\":\"foundation.moist_air.moist_air\"},{\"id\":\"P\",\"label\":\"P\",\"type\":\"output\"}],\"Top\":[]}"
  Volumetric Flow Rate Sensor (MA) : fl_lib/Moist Air/Sensors/Flow Rate Sensor (MA)  mass_flow_measure=false  volumetric_flow_measure=true  volumetric_flow_conditions=foundation.enum.volumetric_flow_conditions.actual  p_std=0.101325 MPa  T_std=20 degC  RH_std=0.65  energy_flow_measure=false  vapor_flow_measure=false  gas_flow_measure=false  droplets_flow_measure=false
      settings: InternalSimscapePortConfiguration="{\"Bottom\":[],\"Left\":[{\"id\":\"A\",\"label\":\"A\",\"type\":\"foundation.moist_air.moist_air\"}],\"Right\":[{\"id\":\"B\",\"label\":\"B\",\"type\":\"foundation.moist_air.moist_air\"},{\"id\":\"V\",\"label\":\"V\",\"type\":\"output\"}],\"Top\":[]}"
  A_P : PMIOPort  Side=Left
  A : PMIOPort  Port=2  Side=Left
  B : PMIOPort  Port=3  Side=Right
  Power : Outport
  wires:
  Abs/1 -> Power/1
  PS-Simulink Converter/1 -> Abs/1
  connections:
  Volumetric Flow Rate Sensor (MA)/LConn1 -- A/RConn1
  Pressure & Temperature Sensor (MA)/LConn1 -- A_P/RConn1
  PS-Simulink Converter/LConn1 -- PS Divide/RConn1
  Average Efficiency/RConn1 -- PS Divide/LConn2
  PS Divide/LConn1 -- PS Product/RConn1
  Volumetric Flow Rate Sensor (MA)/RConn2 -- PS Product/LConn2
  Pressure & Temperature Sensor (MA)/RConn2 -- PS Product/LConn1
  B/RConn1 -- Pressure & Temperature Sensor (MA)/RConn1 -- Volumetric Flow Rate Sensor (MA)/RConn1

== system SSCFuelCell/Recirculation/Feedforward Control ==
  i : Inport
  Constant : Constant  Value=0.2
  Gain : Gain  Gain=0.8 / (stack_iL * stack_area)
  Saturation : Saturate  UpperLimit=1  LowerLimit=0
  Sum : Sum  Inputs=|++
  Transfer Fcn : TransferFcn  Denominator=[2 1]
  cmd : Outport
  wires:
  i/1 -> Gain/1
  Transfer Fcn/1 -> cmd/1
  Gain/1 -> Sum/1
  Constant/1 -> Sum/2
  Sum/1 -> Saturation/1
  Saturation/1 -> Transfer Fcn/1
